simulink model "ThreePhase_Inverter_THI_SPWM"  (R2023a)
settings: Solver=ode23t  StartTime=0.0  StopTime=0.1  MaxStep=1e-4  RelTol=1e-3
libraries: spsMosfetLib x6, simulink x3, spsSeriesRLCBranchLib x3, spsDCVoltageSourceLib x1, spsGroundLib x1, spsThreePhaseVIMeasurementLib x1, sps_lib x1
settings Model: Creator=Alielden  LastModifiedBy=Alielden
settings DataIOCC: SaveState=on  SignalLogging=off  DSMLogging=off  ReturnWorkspaceOutputs=off  LoggingToFile=on

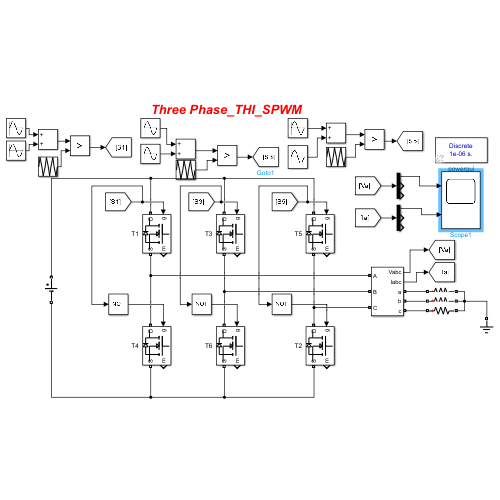
[thumbnail: Simulink's stored preview of the top-level diagram]
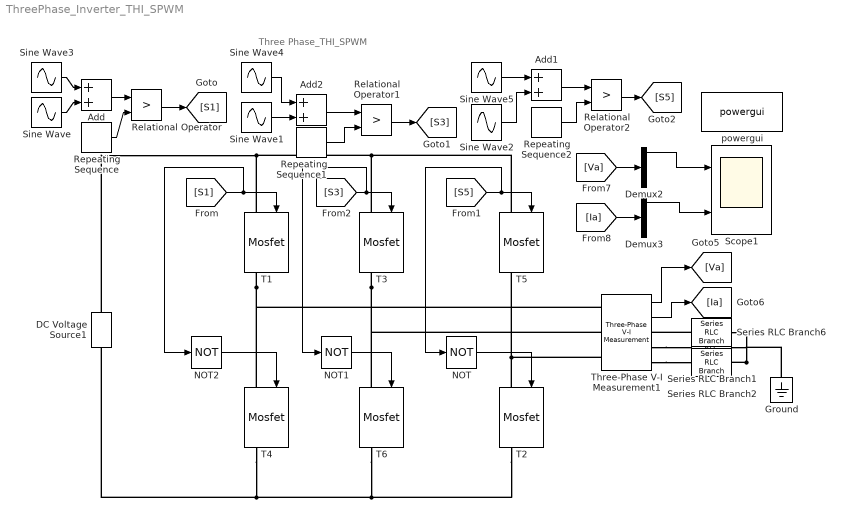
== system ThreePhase_Inverter_THI_SPWM ==
  note: Three Phase_THI_SPWM
  Add : Sum
  Add1 : Sum
  Add2 : Sum
  DC Voltage Source1 : spsDCVoltageSourceLib/DC Voltage Source  Amplitude=100  Measurements=None
  Demux2 : Demux  Outputs=3
  Demux3 : Demux  Outputs=3
  Ground : spsGroundLib/Ground  LConnTagsString=a
  NOT : Logic  Operator=NOT  AllPortsSameDT=off  OutDataTypeStr=boolean
  NOT1 : Logic  Operator=NOT  AllPortsSameDT=off  OutDataTypeStr=boolean
  NOT2 : Logic  Operator=NOT  AllPortsSameDT=off  OutDataTypeStr=boolean
  Relational Operator : RelationalOperator  Operator=>  OutDataTypeStr=boolean  RndMeth=Simplest  InputSameDT=off
  Relational Operator1 : RelationalOperator  Operator=>  OutDataTypeStr=boolean  RndMeth=Simplest  InputSameDT=off
  Relational Operator2 : RelationalOperator  Operator=>  OutDataTypeStr=boolean  RndMeth=Simplest  InputSameDT=off
  Repeating Sequence : simulink/Sources/Repeating Sequence  rep_seq_t="[0 (1/5000)/4  (1/5000)/2  3*(1/5000)/4  (1/5000)]"  rep_seq_y=[0 1 0 -1 0]
  Repeating Sequence1 : simulink/Sources/Repeating Sequence  rep_seq_t="[0 (1/5000)/4  (1/5000)/2  3*(1/5000)/4  (1/5000)]"  rep_seq_y=[0 1 0 -1 0]
  Repeating Sequence2 : simulink/Sources/Repeating Sequence  rep_seq_t="[0 (1/5000)/4  (1/5000)/2  3*(1/5000)/4  (1/5000)]"  rep_seq_y=[0 1 0 -1 0]
  Scope1 : Scope  NumInputPorts=2
  Series RLC Branch1 : spsSeriesRLCBranchLib/Series RLC Branch  LConnTagsString=__new0  RConnTagsString=__new0  BranchType=R  Resistance=10  Inductance=1e-3  SetiL0=off  InitialCurrent=0  Capacitance=1e-6  Setx0=off  InitialVoltage=0  Measurements=None
  Series RLC Branch2 : spsSeriesRLCBranchLib/Series RLC Branch  LConnTagsString=__new0  RConnTagsString=__new0  BranchType=R  Resistance=10  Inductance=1e-3  SetiL0=off  InitialCurrent=0  Capacitance=1e-6  Setx0=off  InitialVoltage=0  Measurements=None
  Series RLC Branch6 : spsSeriesRLCBranchLib/Series RLC Branch  LConnTagsString=__new0  RConnTagsString=__new0  BranchType=R  Resistance=10  Inductance=1e-3  SetiL0=off  InitialCurrent=0  Capacitance=1e-6  Setx0=off  InitialVoltage=0  Measurements=None
  Sine Wave : Sin  Amplitude=1.15  Frequency=100*pi  SampleTime=0
  Sine Wave1 : Sin  Amplitude=1.15  Frequency=100*pi  Phase=120*pi/180  SampleTime=0
  Sine Wave2 : Sin  Amplitude=1.15  Frequency=100*pi  Phase=240*pi/180  SampleTime=0
  Sine Wave3 : Sin  Amplitude=0.19  Frequency=100*pi*3  SampleTime=0
  Sine Wave4 : Sin  Amplitude=0.19  Frequency=100*pi*3  Phase=120*pi/180  SampleTime=0
  Sine Wave5 : Sin  Amplitude=0.19  Frequency=100*pi*3  Phase=240*pi/180  SampleTime=0
  T{1..6} (6 alike) : spsMosfetLib/Mosfet  Ron=0.1  Lon=0  Rd=0.01  Vfd=0  IC=0  Rs=1e5  Cs=inf  Measurements=on
  Three-Phase V-I Measurement1 : spsThreePhaseVIMeasurementLib/Three-Phase V-I Measurement  VoltageMeasurement=phase-to-ground  SetLabelV=off  LabelV=Van  Vpu=off  VpuLL=off  CurrentMeasurement=yes  SetLabelI=off  LabelI=Iabc  Ipu=off  Pbase=100e6  Vbase=500e3  OutputType=Complex  PhasorSimulation=off  PSBequivalent=0
  powergui : sps_lib/powergui  Priority=1  SimulationMode=Discrete  SampleTime=1e-6  frequency=60  Iterations=50  frequencyindice=0  Pbase=100e6  ErrMax=1e-4  UnitsV=kV  UnitsW=MW  buscounter=0  FunctionMessages=off  echomessages=off  EnableUseOfTLC=off  CurrentSourceSwitches=off  DisableSnubberDevices=off  DisableRonSwitches=off  DisableVfSwitches=off  DisplayEquations=off  AutomaticDiscreteSolvers=off  SolverType=Tustin/Backward Euler (TBE)  Interpol=off  ExternalGateDelay=off  methode=off  Ts=100  x0status=blocks  SPID=on  SwTol=0  HookPort=off  NonlinearTolerance=1e-4  nMaxIteration=100  ContinueOnMaxIteration=off  RestoreLinks=warning  ResistiveCurrentMeasurement=off  Frange=[0:2:500]  Ylog=off  Xlog=on  ShowGrid=off  save=off  variable=ZData  structure=0  ZoomFFT=off  StartTime=0.0  cycles=1  DisplayStyle=1  fundamental=60  FreqAxis=off  MaxFrequency=1000  frequencyindicesteady=1  RmsSteady=1  display=off
  wires:
  [S5] -> NOT/1, T5/1
  Relational Operator/1 -> [S1]
  NOT/1 -> T2/1
  [S1] -> NOT2/1, T1/1
  Repeating Sequence/1 -> Relational Operator/2
  Repeating Sequence1/1 -> Relational Operator1/2
  Relational Operator2/1 -> [S5]
  [S3] -> NOT1/1, T3/1
  NOT2/1 -> T4/1
  Relational Operator1/1 -> [S3]
  Repeating Sequence2/1 -> Relational Operator2/2
  NOT1/1 -> T6/1
  Sine Wave3/1 -> Add/1
  Sine Wave/1 -> Add/2
  Add/1 -> Relational Operator/1
  Sine Wave4/1 -> Add2/1
  Sine Wave1/1 -> Add2/2
  Add2/1 -> Relational Operator1/1
  Add1/1 -> Relational Operator2/1
  Sine Wave2/1 -> Add1/2
  Sine Wave5/1 -> Add1/1
  Demux2/1 -> Scope1/1
  Demux3/1 -> Scope1/2
  [Va] -> Demux2/1
  [Ia] -> Demux3/1
  Three-Phase V-I Measurement1/2 -> [Ia]
  Three-Phase V-I Measurement1/1 -> [Va]
  connections:
  T3/LConn1 -- DC Voltage Source1/RConn1 -- T1/LConn1 -- T5/LConn1
  T6/RConn1 -- T2/RConn1 -- DC Voltage Source1/LConn1 -- T4/RConn1
  T3/RConn1 -- T6/LConn1 -- Three-Phase V-I Measurement1/LConn2
  T1/RConn1 -- T4/LConn1 -- Three-Phase V-I Measurement1/LConn1
  Three-Phase V-I Measurement1/LConn3 -- T5/RConn1 -- T2/LConn1
  Series RLC Branch2/RConn1 -- Series RLC Branch6/RConn1 -- Ground/LConn1 -- Series RLC Branch1/RConn1
  Three-Phase V-I Measurement1/RConn2 -- Series RLC Branch1/LConn1
  Three-Phase V-I Measurement1/RConn3 -- Series RLC Branch2/LConn1
  Series RLC Branch6/LConn1 -- Three-Phase V-I Measurement1/RConn1
